simulink model "speedcontroller_rfocim"  (R2019a)
settings: Solver=VariableStepAuto  StartTime=0.0  StopTime=10  RelTol=1e-3
settings Model: Creator=ancem  LastModifiedBy=ancem

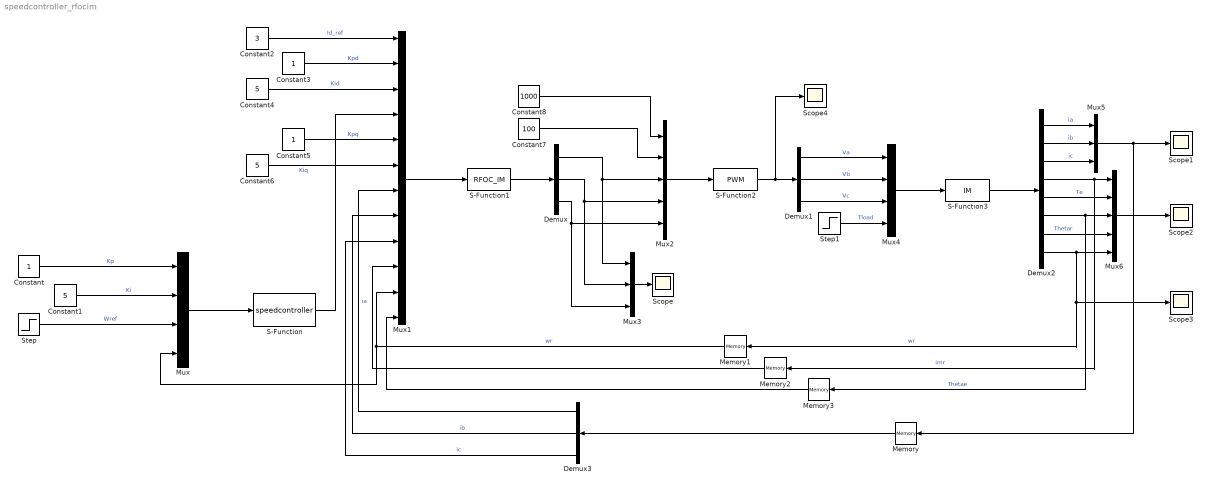
== system speedcontroller_rfocim ==
  Constant : Constant
  Constant1 : Constant  Value=5
  Constant2 : Constant  Value=3
  Constant3 : Constant
  Constant4 : Constant  Value=5
  Constant5 : Constant
  Constant6 : Constant  Value=5
  Constant7 : Constant  Value=100
  Constant8 : Constant  Value=1000
  Demux : Demux  Outputs=3
  Demux1 : Demux  Outputs=3
  Demux2 : Demux  Outputs=8
  Demux3 : Demux  Outputs=3
  Memory{,1..3} (4 alike) : Memory
  Mux : Mux
  Mux1 : Mux  Inputs=12
  Mux2 : Mux  Inputs=5
  Mux3 : Mux  Inputs=3
  Mux4 : Mux
  Mux5 : Mux  Inputs=3
  Mux6 : Mux  Inputs=5
  S-Function : S-Function  FunctionName=speedcontroller  SFunctionDeploymentMode=off  EnableBusSupport=off
  S-Function1 : S-Function  FunctionName=RFOC_IM  SFunctionDeploymentMode=off  EnableBusSupport=off
  S-Function2 : S-Function  FunctionName=PWM  SFunctionDeploymentMode=off  EnableBusSupport=off
  S-Function3 : S-Function  FunctionName=IM  SFunctionDeploymentMode=off  EnableBusSupport=off
  Scope{,1..4} (5 alike) : Scope
  Step : Step  After=10  SampleTime=0
  Step1 : Step  Time=3  After=2  SampleTime=0
  wires:
  Mux/1 -> S-Function/1
  Constant/1 -> Mux/1  "Kp"
  Constant1/1 -> Mux/2  "Ki"
  Step/1 -> Mux/3  "Wref"
  Mux1/1 -> S-Function1/1
  S-Function/1 -> Mux1/4
  Constant2/1 -> Mux1/1  "Id_ref"
  Constant3/1 -> Mux1/2  "Kpd"
  Constant4/1 -> Mux1/3  "Kid"
  Constant5/1 -> Mux1/5  "Kpq"
  Constant6/1 -> Mux1/6  "Kiq"
  S-Function1/1 -> Demux/1
  Mux2/1 -> S-Function2/1
  Demux/1 -> Mux2/3, Mux3/1
  Demux/2 -> Mux3/2, Mux2/4
  Demux/3 -> Mux3/3, Mux2/5
  Mux3/1 -> Scope/1
  Constant7/1 -> Mux2/2
  Constant8/1 -> Mux2/1
  S-Function2/1 -> Scope4/1, Demux1/1
  Demux1/1 -> Mux4/1  "Va"
  Demux1/2 -> Mux4/2  "Vb"
  Demux1/3 -> Mux4/3  "Vc"
  Step1/1 -> Mux4/4  "Tload"
  Mux4/1 -> S-Function3/1
  S-Function3/1 -> Demux2/1
  Demux2/1 -> Mux5/1  "ia"
  Demux2/2 -> Mux5/2  "ib"
  Demux2/3 -> Mux5/3  "ic"
  Mux5/1 -> Memory/1, Scope1/1
  Demux2/4 -> Memory2/1, Mux6/1  "imr"
  Demux2/5 -> Mux6/2  "Te"
  Demux2/6 -> Mux6/3, Memory3/1  "Thetae"
  Demux2/7 -> Mux6/4  "Thetar"
  Demux2/8 -> Mux6/5, Scope3/1, Memory1/1  "wr"
  Mux6/1 -> Scope2/1
  Memory/1 -> Demux3/1
  Demux3/1 -> Mux1/7  "ia"
  Demux3/2 -> Mux1/8  "ib"
  Demux3/3 -> Mux1/9  "ic"
  Memory1/1 -> Mux/4, Mux1/11  "wr"
  Memory2/1 -> Mux1/10
  Memory3/1 -> Mux1/12
